simulink model "untitled"  (R2024a)
settings: Solver=FixedStepDiscrete  StartTime=0  StopTime=10.0  RelTol=1e-3
settings Model: Creator=aero  LastModifiedBy=aero
settings OptimizationCC: DefaultParameterBehavior=Inlined  EnhancedBackFolding=on  PassReuseOutputArgsAs=Individual arguments  ZeroExternalMemoryAtStartup=off  ZeroInternalMemoryAtStartup=off  OptimizeBlockOrder=speed  DifferentSizesBufferReuse=on  OptimizationCustomize=off  EfficientTunableParamExpr=on
settings DebuggingCC: ParameterTunabilityLossMsg=error
settings SFSimCC: MATLABDynamicMemAlloc=off  SimTargetLang=C++
settings RTWCC: Description=Embedded Coder  SystemTargetFile=ert.tlc  TemplateMakefile=ert_default_tmf  TargetLang=C++
settings CodeAppCC: ForceParamTrailComments=on  IgnoreCustomStorageClasses=off  OperatorAnnotations=on  SimulinkDataObjDesc=on  SFDataObjDesc=on  InsertBlockDesc=on
settings ERTTargetCC: TargetLangStandard=C++11 (ISO)  GenerateSampleERTMain=on  CodeInterfacePackaging=C++ class  InlinedParameterPlacement=NonHierarchical  RootIOFormat=Structure reference  ERTCustomFileTemplate=example_file_process.tlc

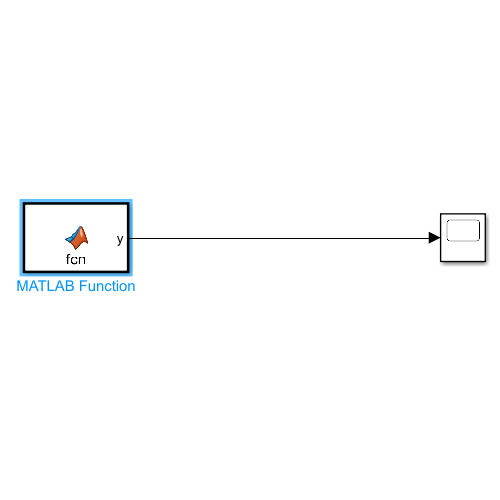
[thumbnail: Simulink's stored preview of the top-level diagram]
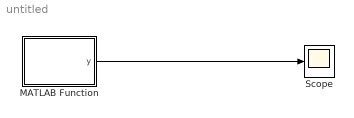
== system untitled ==
  MATLAB Function : MATLAB Function  TreatAsAtomicUnit=on
  Scope : Scope
  wires:
  MATLAB Function/1(y) -> Scope/1

== matlab function untitled/MATLAB Function ==
  data: y output
function y = fcn()

A1 = [eye(2); -eye(2)];
b1 = [5; 5; 5; 5];

A = api.Polyhedron(A1, b1);

A2 = [-eye(2); eye(2)];
b2 = [1; 1; 1; 1];

B = api.Polyhedron(A2, b2);

contained = api.Contains(A, B)

S = api.Minus(A, B);

y = 10;
